simulink model "PruebaTOC"  (R2025a)
settings: Solver=FixedStepDiscrete  StartTime=0.0  StopTime=inf  FixedStep=0.01  RelTol=1e-3  EnableMultiTasking=on
libraries: arduinolib x10, svdutilitieslib x3, arduinosensorlib x2
settings Model: SILPILModeSetting=veronly  ExtModeTrigDuration=2  Creator=aj  LastModifiedBy=aj
settings SolverCC: AutoInsertRateTranBlk=on
settings OptimizationCC: EnhancedBackFolding=on  PassReuseOutputArgsAs=Individual arguments  ZeroExternalMemoryAtStartup=off  ZeroInternalMemoryAtStartup=off  MaxStackSize=64  OptimizeBlockOrder=speed  DifferentSizesBufferReuse=on  OptimizationCustomize=off  EfficientTunableParamExpr=on
settings DebuggingCC: ParameterTunabilityLossMsg=error
settings HardwareCC: ProdBitPerPointer=32.0  ProdBitPerSizeT=32.0  ProdBitPerPtrDiffT=32.0  ProdLargestAtomicInteger=Long  ProdLargestAtomicFloat=Double  ProdWordSize=32.0  ProdHWDeviceType=ARM Compatible->ARM Cortex
settings SFSimCC: MATLABDynamicMemAlloc=off
settings RTWCC: SystemTargetFile=ert.tlc  HardwareBoard=ESP32-WROOM (Arduino Compatible)  TLCOptions="-aInlineSetEventsForThisBaseRateFcn=TLC_FALSE -aSuppressMultiTaskScheduler=TLC_FALSE  -aRateBasedStepFcn=0"  TemplateMakefile=ert_default_tmf  Toolchain=ESP32  BuildConfiguration=Faster Runs  Description=Embedded Coder
settings CodeAppCC: ForceParamTrailComments=on  IgnoreCustomStorageClasses=off  OperatorAnnotations=on  SimulinkDataObjDesc=on  SFDataObjDesc=on  InsertBlockDesc=on
settings ERTTargetCC: ExtModeTransport=3.0  ExtModeAutomaticAllocSize=off  ExtModeStaticAllocSize=65536.0  InlinedParameterPlacement=Hierarchical  SupportContinuousTime=on  SupportVariableSizeSignals=on

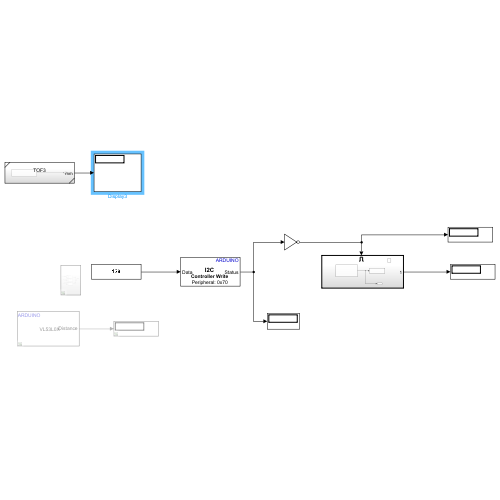
[thumbnail: Simulink's stored preview of the top-level diagram]
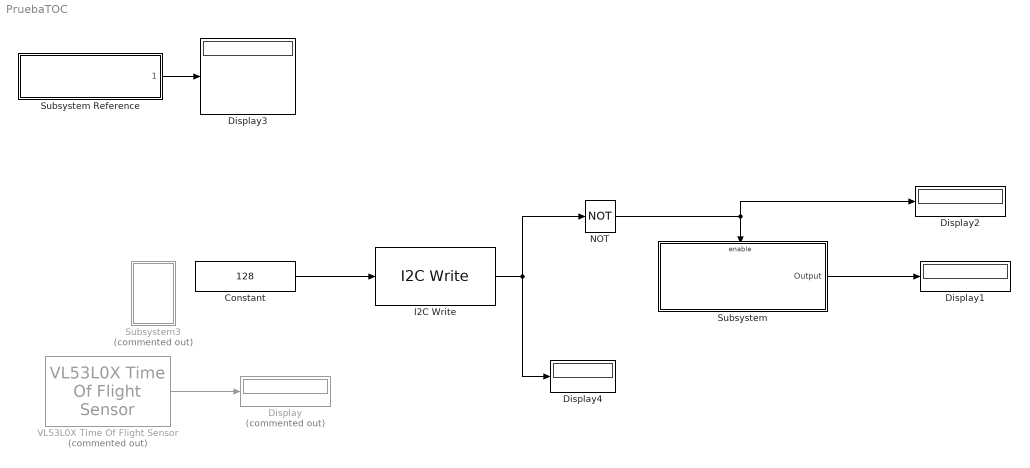
== system PruebaTOC ==
  Constant : Constant  Value=128  OutDataTypeStr=uint8  SampleTime=.05
  Display : Display  Commented=on
  Display{1..4} (4 alike) : Display
  I2C Write : arduinolib/I2C Write  I2CModule=0  Mode=Master  SlaveAddress=0x70  SlaveByteOrder=BigEndian  Direction=Transmitter  RegisterAddressMode=off  RegisterAddress=0  SlaveDataType=uint8  DataLength=1  NoAck=off  RepeatedStart=off  OutputStatus=on  blockPlatform=ARDUINO
  NOT : Logic  Operator=NOT  IconShape=distinctive  AllPortsSameDT=off  OutDataTypeStr=boolean
  Subsystem : Subsystem
  Subsystem Reference : Subsystem  ReferencedSubsystem=TOF3
  Subsystem3 : Subsystem  Commented=on
  VL53L0X Time Of Flight Sensor : arduinosensorlib/VL53L0X Time Of Flight Sensor  Commented=on  I2CModule=0  I2CAddress=0x29  BitRate=1000000  RangingMode=Default  SampleTime=0.05
  wires:
  VL53L0X Time Of Flight Sensor/1 -> Display/1
  NOT/1 -> Subsystem/Enable, Display2/1
  Constant/1 -> I2C Write/1
  I2C Write/1 -> NOT/1, Display4/1
  Subsystem/1(Output) -> Display1/1
  Subsystem Reference/1 -> Display3/1

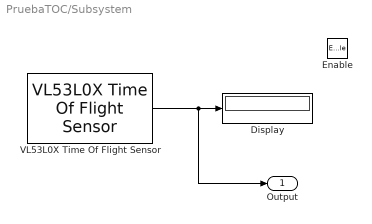
== system PruebaTOC/Subsystem ==
  Enable : EnablePort
  Display : Display
  VL53L0X Time Of Flight Sensor : arduinosensorlib/VL53L0X Time Of Flight Sensor  I2CModule=0  I2CAddress=0x29  BitRate=1000000  RangingMode=Default  SampleTime=0.05
  Output : Outport
  wires:
  VL53L0X Time Of Flight Sensor/1 -> Output/1, Display/1

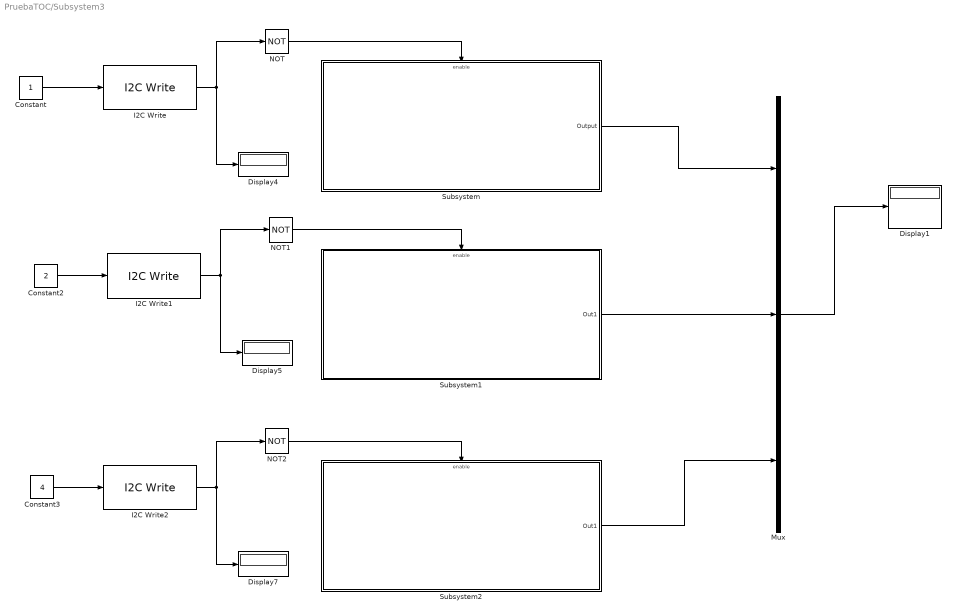
== system PruebaTOC/Subsystem3 ==
  Constant : Constant  OutDataTypeStr=uint8
  Constant2 : Constant  Value=2  OutDataTypeStr=uint8
  Constant3 : Constant  Value=4  OutDataTypeStr=uint8
  Display{1,4..5,7} (4 alike) : Display
  I2C Write : arduinolib/I2C Write  I2CModule=0  Mode=Master  SlaveAddress=0x70  SlaveByteOrder=BigEndian  Direction=Transmitter  RegisterAddressMode=off  RegisterAddress=0  SlaveDataType=uint8  DataLength=1  NoAck=off  RepeatedStart=off  OutputStatus=on  blockPlatform=ARDUINO
  I2C Write1 : arduinolib/I2C Write  I2CModule=0  Mode=Master  SlaveAddress=0x70  SlaveByteOrder=BigEndian  Direction=Transmitter  RegisterAddressMode=off  RegisterAddress=0  SlaveDataType=uint8  DataLength=1  NoAck=off  RepeatedStart=off  OutputStatus=on  blockPlatform=ARDUINO
  I2C Write2 : arduinolib/I2C Write  I2CModule=0  Mode=Master  SlaveAddress=0x70  SlaveByteOrder=BigEndian  Direction=Transmitter  RegisterAddressMode=off  RegisterAddress=0  SlaveDataType=uint8  DataLength=1  NoAck=off  RepeatedStart=off  OutputStatus=on  blockPlatform=ARDUINO
  Mux : Mux  Inputs=3
  NOT : Logic  Operator=NOT  IconShape=distinctive  AllPortsSameDT=off  OutDataTypeStr=boolean
  NOT1 : Logic  Operator=NOT  IconShape=distinctive  AllPortsSameDT=off  OutDataTypeStr=boolean
  NOT2 : Logic  Operator=NOT  IconShape=distinctive  AllPortsSameDT=off  OutDataTypeStr=boolean
  Subsystem : Subsystem
  Subsystem1 : Subsystem
  Subsystem2 : Subsystem
  wires:
  Mux/1 -> Display1/1
  I2C Write/1 -> NOT/1, Display4/1
  Subsystem2/1(Out1) -> Mux/3
  Subsystem/1(Output) -> Mux/1
  I2C Write2/1 -> NOT2/1, Display7/1
  Constant/1 -> I2C Write/1
  I2C Write1/1 -> NOT1/1, Display5/1
  NOT/1 -> Subsystem/Enable
  Constant2/1 -> I2C Write1/1
  Subsystem1/1(Out1) -> Mux/2
  NOT1/1 -> Subsystem1/Enable
  NOT2/1 -> Subsystem2/Enable
  Constant3/1 -> I2C Write2/1

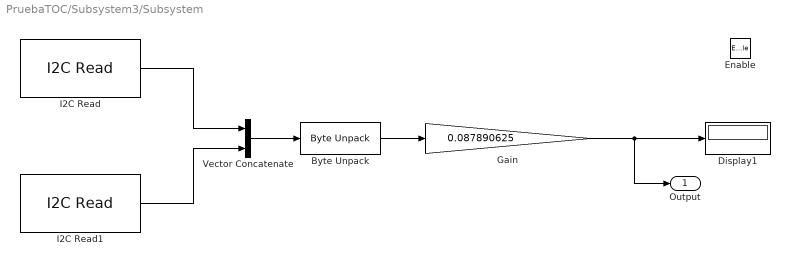
== system PruebaTOC/Subsystem3/Subsystem ==
  Enable : EnablePort
  Byte Unpack : svdutilitieslib/Byte Unpack  dimensions={[1]}  datatypes={'int16'}  byteAlign=1  blockPlatform=arduinoert
  Display1 : Display
  Gain : Gain  Gain=0.087890625
  I2C Read : arduinolib/I2C Read  I2CModule=0  Mode=Master  SlaveAddress=54  SlaveByteOrder=BigEndian  Direction=Receiver  RegisterAddressMode=on  RegisterAddress=13  SlaveDataType=uint8  DataLength=1  NoAck=off  RepeatedStart=off  OutputStatus=off  blockPlatform=ARDUINO  SampleTime=0.01
  I2C Read1 : arduinolib/I2C Read  I2CModule=0  Mode=Master  SlaveAddress=54  SlaveByteOrder=BigEndian  Direction=Receiver  RegisterAddressMode=on  RegisterAddress=12  SlaveDataType=uint8  DataLength=1  NoAck=off  RepeatedStart=off  OutputStatus=off  blockPlatform=ARDUINO  SampleTime=0.01
  Vector Concatenate : Concatenate
  Output : Outport
  wires:
  Vector Concatenate/1 -> Byte Unpack/1
  I2C Read/1 -> Vector Concatenate/1
  I2C Read1/1 -> Vector Concatenate/2
  Byte Unpack/1 -> Gain/1
  Gain/1 -> Output/1, Display1/1

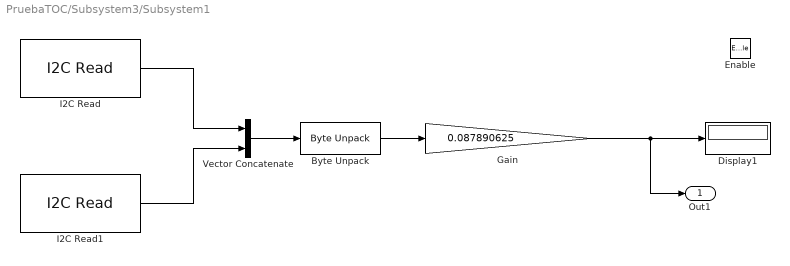
== system PruebaTOC/Subsystem3/Subsystem1 ==
  Enable : EnablePort
  Byte Unpack : svdutilitieslib/Byte Unpack  dimensions={[1]}  datatypes={'int16'}  byteAlign=1  blockPlatform=arduinoert
  Display1 : Display
  Gain : Gain  Gain=0.087890625
  I2C Read : arduinolib/I2C Read  I2CModule=0  Mode=Master  SlaveAddress=54  SlaveByteOrder=BigEndian  Direction=Receiver  RegisterAddressMode=on  RegisterAddress=13  SlaveDataType=uint8  DataLength=1  NoAck=off  RepeatedStart=off  OutputStatus=off  blockPlatform=ARDUINO  SampleTime=0.01
  I2C Read1 : arduinolib/I2C Read  I2CModule=0  Mode=Master  SlaveAddress=54  SlaveByteOrder=BigEndian  Direction=Receiver  RegisterAddressMode=on  RegisterAddress=12  SlaveDataType=uint8  DataLength=1  NoAck=off  RepeatedStart=off  OutputStatus=off  blockPlatform=ARDUINO  SampleTime=0.01
  Vector Concatenate : Concatenate
  Out1 : Outport
  wires:
  Vector Concatenate/1 -> Byte Unpack/1
  I2C Read/1 -> Vector Concatenate/1
  I2C Read1/1 -> Vector Concatenate/2
  Byte Unpack/1 -> Gain/1
  Gain/1 -> Out1/1, Display1/1

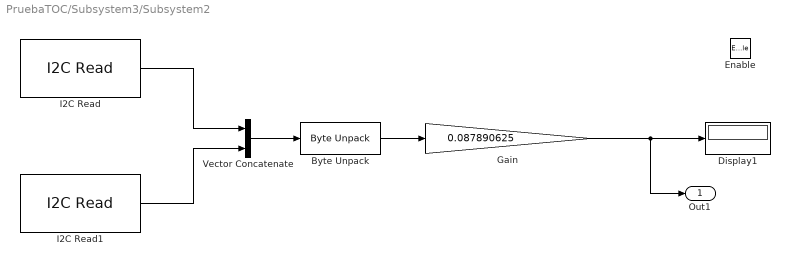
== system PruebaTOC/Subsystem3/Subsystem2 ==
  Enable : EnablePort
  Byte Unpack : svdutilitieslib/Byte Unpack  dimensions={[1]}  datatypes={'int16'}  byteAlign=1  blockPlatform=arduinoert
  Display1 : Display
  Gain : Gain  Gain=0.087890625
  I2C Read : arduinolib/I2C Read  I2CModule=0  Mode=Master  SlaveAddress=54  SlaveByteOrder=BigEndian  Direction=Receiver  RegisterAddressMode=on  RegisterAddress=13  SlaveDataType=uint8  DataLength=1  NoAck=off  RepeatedStart=off  OutputStatus=off  blockPlatform=ARDUINO  SampleTime=0.01
  I2C Read1 : arduinolib/I2C Read  I2CModule=0  Mode=Master  SlaveAddress=54  SlaveByteOrder=BigEndian  Direction=Receiver  RegisterAddressMode=on  RegisterAddress=12  SlaveDataType=uint8  DataLength=1  NoAck=off  RepeatedStart=off  OutputStatus=off  blockPlatform=ARDUINO  SampleTime=0.01
  Vector Concatenate : Concatenate
  Out1 : Outport
  wires:
  Vector Concatenate/1 -> Byte Unpack/1
  I2C Read/1 -> Vector Concatenate/1
  I2C Read1/1 -> Vector Concatenate/2
  Byte Unpack/1 -> Gain/1
  Gain/1 -> Out1/1, Display1/1
